simulink model "sampleModel7293_pp_1_1_mu"  (R2018a)
settings: Solver=VariableStepAuto  StartTime=0.0  StopTime=10.0  RelTol=1e-3
undefined symbols (not defined in the file): DiscIntNeverNeededParam
libraries: simulink x367
(part 1 of 13)
settings Model: Creator=cyfuzz  LastModifiedBy=shafiul
settings CodeAppCC: StateflowObjectComments=on

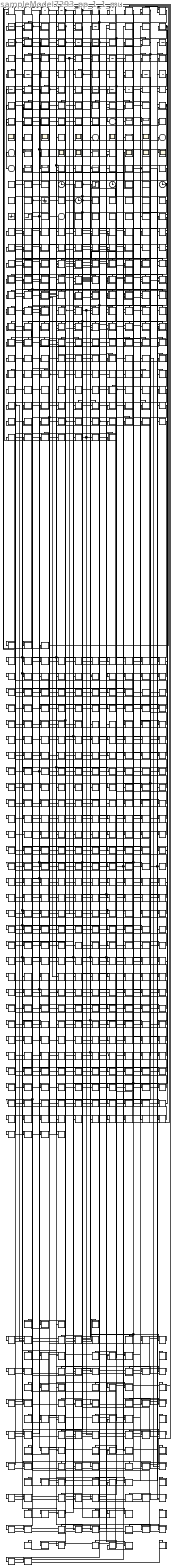
== system sampleModel7293_pp_1_1_mu ==
  cfblk134 : Inport
  cfblk{1,59..60,67} (4 alike) : simulink/Continuous/PID Controller (2DOF)  Controller=PID  TimeDomain=Discrete-time  SampleTime=1  IntegratorMethod=Forward Euler  FilterMethod=Forward Euler  Form=Parallel  UseFilter=on  ControllerParametersSource=internal  P=1  I=1  D=0  N=100  b=1  c=1  InitialConditionSource=internal  InitialConditionForIntegrator=0  InitialConditionForFilter=0  ExternalReset=none  LimitOutput=off  UpperSaturationLimit=inf  LowerSaturationLimit=-inf  LinearizeAsGain=off  AntiWindupMode=none  Kb=1  TrackingMode=off  Kt=1  PParamMin=[]  PParamMax=[]  IParamMin=[]  IParamMax=[]  DParamMin=[]  DParamMax=[]  NParamMin=[]  NParamMax=[]  bParamMin=[]  bParamMax=[]  cParamMin=[]  cParamMax=[]  KbParamMin=[]  KbParamMax=[]  KtParamMin=[]  KtParamMax=[]  POutMin=[]  POutMax=[]  IOutMin=[]  IOutMax=[]  DOutMin=[]  DOutMax=[]  NOutMin=[]  NOutMax=[]  bOutMin=[]  bOutMax=[]  cOutMin=[]  cOutMax=[]  KbOutMin=[]  KbOutMax=[]  KtOutMin=[]  KtOutMax=[]  IntegratorOutMin=[]  IntegratorOutMax=[]  FilterOutMin=[]  FilterOutMax=[]  SumOutMin=[]  SumOutMax=[]  Sum1OutMin=[]  Sum1OutMax=[]  Sum2OutMin=[]  Sum2OutMax=[]  Sum3OutMin=[]  Sum3OutMax=[]  SumI1OutMin=[]  SumI1OutMax=[]  SumI2OutMin=[]  SumI2OutMax=[]  SumI3OutMin=[]  SumI3OutMax=[]  SumDOutMin=[]  SumDOutMax=[]  SaturationOutMin=[]  SaturationOutMax=[]  IntegratorContinuousStateAttributes=''  IntegratorStateMustResolveToSignalObject=off  IntegratorRTWStateStorageClass=Auto  FilterContinuousStateAttributes=''  FilterStateMustResolveToSignalObject=off  FilterRTWStateStorageClass=Auto  DifferentiatorICPrevScaledInput=0  DifferentiatorOutMin=[]  DifferentiatorOutMax=[]  FilterDiffOutCoefMin=[]  FilterDiffOutCoefMax=[]  SumDenOutMin=[]  SumDenOutMax=[]  SumNumOutMin=[]  SumNumOutMax=[]  ReciprocalOutMin=[]  ReciprocalOutMax=[]  DivideOutMin=[]  DivideOutMax=[]  TunerSelectOption=Transfer Function Based (PID Tuner App)
  cfblk{10,15,35,48,54,70,73} (7 alike) : Delay  ShowEnablePort=on  SampleTime=1
      settings: InputPortMap=u0,e6
  cfblk{81,83,85,87,89,94..95,98..100} (10 alike) : Scope
      cfblk81 settings: Floating=on
      cfblk83 settings: Floating=on
      cfblk85 settings: Floating=on
      cfblk87 settings: Floating=on
      cfblk89 settings: Floating=on
      cfblk94 settings: Floating=on
      cfblk95 settings: Floating=on
      cfblk99 settings: Floating=on
  cfblk{78..79,88,92,96,102..103,106} (8 alike) : Display
  cfblk104 : simulink/Sinks/XY Graph  xmin=-1  xmax=1  ymin=-1  ymax=1  st=-1
  cfblk105 : ToWorkspace  VariableName=oefgltt  SaveFormat=Timeseries  SampleTime=-1
  cfblk107 : ToWorkspace  VariableName=romnstx  SaveFormat=Timeseries  SampleTime=-1
  cfblk{108..109,129..130} (4 alike) : RandomNumber  SampleTime=0.1
  cfblk{11,21,26,56} (4 alike) : DiscreteFilter  SampleTime=1
  cfblk110 : simulink/Sources/Counter Limited  uplimit=7  tsamp=1
  cfblk111 : simulink/Sources/Counter Free-Running  NumBits=16  tsamp=1
  cfblk112 : simulink/Sources/Ramp  slope=1  start=0  InitialOutput=0
  cfblk113 : simulink/Sources/Repeating Sequence Interpolated  OutValues=[3 1 4 2 1].'  TimeValues=[0 0.1 0.5 0.6 1].'  LookUpMeth=Interpolation-Use End Values  tsamp=0.01  OutMin=[]  OutMax=[]  OutDataTypeStr=double  OutputDataTypeScalingMode=double  OutDataType=fixdt(0,8)  OutScaling=2^-10
  cfblk{114,117,120,125} (4 alike) : Clock
  cfblk115 : DigitalClock
  cfblk116 : Step  After=79  SampleTime=0
  cfblk118 : simulink/Sources/Counter Free-Running  NumBits=16  tsamp=1
  cfblk119 : simulink/Sources/Repeating Sequence  rep_seq_t=[0 2]  rep_seq_y=[0 2]
  cfblk12 : Subsystem  TreatAsAtomicUnit=on
  cfblk121 : simulink/Sources/Repeating Sequence Stair  OutValues=[3 1 4 2 1].'  tsamp=1  OutMin=[]  OutMax=[]  OutDataTypeStr=double  OutputDataTypeScalingMode=double  OutDataType=fixdt(0,8)  ConRadixGroup=Best Precision: Vector-wise  OutScaling=2^-12
  cfblk122 : Constant  Value=5474  OutDataTypeStr=double  SampleTime=1
  cfblk123 : Ground
  cfblk124 : simulink/Sources/Chirp Signal  f1=0.1  T=100  f2=1
  cfblk126 : Constant  Value=0696  OutDataTypeStr=double  SampleTime=1
  cfblk127 : simulink/Sources/Repeating Sequence Stair  OutValues=[3 1 4 2 1].'  tsamp=1  OutMin=[]  OutMax=[]  OutDataTypeStr=double  OutputDataTypeScalingMode=double  OutDataType=fixdt(0,8)  ConRadixGroup=Best Precision: Vector-wise  OutScaling=2^-12
  cfblk128 : SignalGenerator  Units=rad/sec
  cfblk{13,23,46,65,216..217,221..226,228..229,232,234..238,241..246,248..254,257..258,260..267,269..272} (47 alike) : Delay  SampleTime=1
  cfblk131 : Ground
  cfblk132 : Step  After=47  SampleTime=0
  cfblk133 : simulink/Sources/Counter Limited  uplimit=7  tsamp=1
  cfblk135 : simulink/Sources/Repeating Sequence Stair  OutValues=[3 1 4 2 1].'  tsamp=1  OutMin=[]  OutMax=[]  OutDataTypeStr=double  OutputDataTypeScalingMode=double  OutDataType=fixdt(0,8)  ConRadixGroup=Best Precision: Vector-wise  OutScaling=2^-12
  cfblk136 : simulink/Sources/Repeating Sequence Interpolated  OutValues=[3 1 4 2 1].'  TimeValues=[0 0.1 0.5 0.6 1].'  LookUpMeth=Interpolation-Use End Values  tsamp=0.01  OutMin=[]  OutMax=[]  OutDataTypeStr=double  OutputDataTypeScalingMode=double  OutDataType=fixdt(0,8)  OutScaling=2^-10
  cfblk137 : DigitalClock
  cfblk138 : simulink/Sources/Repeating Sequence Interpolated  OutValues=[3 1 4 2 1].'  TimeValues=[0 0.1 0.5 0.6 1].'  LookUpMeth=Interpolation-Use End Values  tsamp=0.01  OutMin=[]  OutMax=[]  OutDataTypeStr=double  OutputDataTypeScalingMode=double  OutDataType=fixdt(0,8)  OutScaling=2^-10
  cfblk{139..163} (25 alike) : If  SampleTime=1
  cfblk14 : DiscreteStateSpace
  cfblk{4,16,25,37,51} (5 alike) : DiscreteIntegrator  OutDataTypeStr=double  ICPrevOutput=DiscIntNeverNeededParam  ICPrevScaledInput=DiscIntNeverNeededParam
  cfblk164 : Subsystem  TreatAsAtomicUnit=on
  cfblk165 : Subsystem  TreatAsAtomicUnit=on
  cfblk166 : Subsystem  TreatAsAtomicUnit=on
  cfblk167 : Subsystem  TreatAsAtomicUnit=on
  cfblk168 : Subsystem  TreatAsAtomicUnit=on
  cfblk169 : Subsystem  TreatAsAtomicUnit=on
  cfblk{17,24,36,43..44,71} (6 alike) : Delay  DelayLengthSource=Input port  SampleTime=1
      settings: InputPortMap=u0,p1
  cfblk170 : Subsystem  TreatAsAtomicUnit=on
  cfblk171 : Subsystem  TreatAsAtomicUnit=on
  cfblk172 : Subsystem  TreatAsAtomicUnit=on
  cfblk173 : Subsystem  TreatAsAtomicUnit=on
  cfblk174 : Subsystem  TreatAsAtomicUnit=on
  cfblk175 : Subsystem  TreatAsAtomicUnit=on
  cfblk176 : Subsystem  TreatAsAtomicUnit=on
  cfblk177 : Subsystem  TreatAsAtomicUnit=on
  cfblk178 : Subsystem  TreatAsAtomicUnit=on
  cfblk179 : Subsystem  TreatAsAtomicUnit=on
  cfblk{18,34,47,69} (4 alike) : simulink/Continuous/PID Controller  Controller=PID  TimeDomain=Discrete-time  SampleTime=1  IntegratorMethod=Forward Euler  FilterMethod=Forward Euler  Form=Parallel  UseFilter=on  ControllerParametersSource=internal  P=1  I=1  D=0  N=100  InitialConditionSource=internal  InitialConditionForIntegrator=0  InitialConditionForFilter=0  ExternalReset=none  LimitOutput=off  UpperSaturationLimit=inf  LowerSaturationLimit=-inf  LinearizeAsGain=off  AntiWindupMode=none  Kb=1  TrackingMode=off  Kt=1  PParamMin=[]  PParamMax=[]  IParamMin=[]  IParamMax=[]  DParamMin=[]  DParamMax=[]  NParamMin=[]  NParamMax=[]  KbParamMin=[]  KbParamMax=[]  KtParamMin=[]  KtParamMax=[]  POutMin=[]  POutMax=[]  IOutMin=[]  IOutMax=[]  DOutMin=[]  DOutMax=[]  NOutMin=[]  NOutMax=[]  KbOutMin=[]  KbOutMax=[]  KtOutMin=[]  KtOutMax=[]  IntegratorOutMin=[]  IntegratorOutMax=[]  FilterOutMin=[]  FilterOutMax=[]  SumOutMin=[]  SumOutMax=[]  SumI1OutMin=[]  SumI1OutMax=[]  SumI2OutMin=[]  SumI2OutMax=[]  SumI3OutMin=[]  SumI3OutMax=[]  SumDOutMin=[]  SumDOutMax=[]  SaturationOutMin=[]  SaturationOutMax=[]  IntegratorContinuousStateAttributes=''  IntegratorStateMustResolveToSignalObject=off  IntegratorRTWStateStorageClass=Auto  FilterContinuousStateAttributes=''  FilterStateMustResolveToSignalObject=off  FilterRTWStateStorageClass=Auto  DifferentiatorICPrevScaledInput=0  DifferentiatorOutMin=[]  DifferentiatorOutMax=[]  FilterDiffOutCoefMin=[]  FilterDiffOutCoefMax=[]  SumDenOutMin=[]  SumDenOutMax=[]  SumNumOutMin=[]  SumNumOutMax=[]  ReciprocalOutMin=[]  ReciprocalOutMax=[]  DivideOutMin=[]  DivideOutMax=[]  TunerSelectOption=Transfer Function Based (PID Tuner App)
  cfblk180 : Subsystem  TreatAsAtomicUnit=on
  cfblk181 : Subsystem  TreatAsAtomicUnit=on
  cfblk182 : Subsystem  TreatAsAtomicUnit=on
  cfblk183 : Subsystem  TreatAsAtomicUnit=on
  cfblk184 : Subsystem  TreatAsAtomicUnit=on
  cfblk185 : Subsystem  TreatAsAtomicUnit=on
  cfblk186 : Subsystem  TreatAsAtomicUnit=on
  cfblk187 : Subsystem  TreatAsAtomicUnit=on
  cfblk188 : Subsystem  TreatAsAtomicUnit=on
  cfblk189 : Subsystem  TreatAsAtomicUnit=on
  cfblk19 : simulink/Discrete/Transfer Fcn Real Zero  ZeroZ=0.75  ICPrevInput=0.0  DoSatur=off
      settings: SourceProductName=Simulink  SourceProductBaseCode=SL
  cfblk190 : Subsystem  TreatAsAtomicUnit=on
  cfblk191 : Subsystem  TreatAsAtomicUnit=on
  cfblk192 : Subsystem  TreatAsAtomicUnit=on
  cfblk193 : Subsystem  TreatAsAtomicUnit=on
  cfblk194 : Subsystem  TreatAsAtomicUnit=on
  cfblk195 : Subsystem  TreatAsAtomicUnit=on
  cfblk196 : Subsystem  TreatAsAtomicUnit=on
  cfblk197 : Subsystem  TreatAsAtomicUnit=on
  cfblk198 : Subsystem  TreatAsAtomicUnit=on
  cfblk199 : Subsystem  TreatAsAtomicUnit=on
  cfblk2 : Subsystem  TreatAsAtomicUnit=on
  cfblk20 : simulink/Discrete/Transfer Fcn First Order  PoleZ=0.95  ICPrevOutput=0.0  DoSatur=off
      settings: SourceProductName=Simulink
  cfblk200 : Subsystem  TreatAsAtomicUnit=on
  cfblk201 : Subsystem  TreatAsAtomicUnit=on
  cfblk202 : Subsystem  TreatAsAtomicUnit=on
  cfblk203 : Subsystem  TreatAsAtomicUnit=on
  cfblk204 : Subsystem  TreatAsAtomicUnit=on
  cfblk205 : Subsystem  TreatAsAtomicUnit=on
  cfblk206 : Subsystem  TreatAsAtomicUnit=on
  cfblk207 : Subsystem  TreatAsAtomicUnit=on
  cfblk208 : Subsystem  TreatAsAtomicUnit=on
  cfblk209 : Subsystem  TreatAsAtomicUnit=on
  cfblk210 : Subsystem  TreatAsAtomicUnit=on
  cfblk211 : Subsystem  TreatAsAtomicUnit=on
  cfblk212 : Subsystem  TreatAsAtomicUnit=on
  cfblk213 : Subsystem  TreatAsAtomicUnit=on
  cfblk214 : Subsystem  TreatAsAtomicUnit=on
  cfblk215 : Subsystem  TreatAsAtomicUnit=on
  cfblk218 : Subsystem  TreatAsAtomicUnit=on
  cfblk219 : Subsystem  TreatAsAtomicUnit=on
  cfblk22 : Subsystem  TreatAsAtomicUnit=on
  cfblk220 : Subsystem  TreatAsAtomicUnit=on
  cfblk227 : Subsystem  TreatAsAtomicUnit=on
  cfblk230 : Subsystem  TreatAsAtomicUnit=on
  cfblk231 : Subsystem  TreatAsAtomicUnit=on
  cfblk233 : Subsystem  TreatAsAtomicUnit=on
  cfblk239 : Subsystem  TreatAsAtomicUnit=on
  cfblk240 : Subsystem  TreatAsAtomicUnit=on
  cfblk247 : Subsystem  TreatAsAtomicUnit=on
  cfblk255 : Subsystem  TreatAsAtomicUnit=on
  cfblk256 : Subsystem  TreatAsAtomicUnit=on
  cfblk259 : Subsystem  TreatAsAtomicUnit=on
  cfblk268 : Subsystem  TreatAsAtomicUnit=on
  cfblk27 : DiscreteZeroPole  Poles=[0 0.5]  Gain=1
  cfblk273 : Subsystem  TreatAsAtomicUnit=on
  cfblk274 : DataTypeConversion  OutDataTypeStr=double
  cfblk275 : DataTypeConversion  OutDataTypeStr=double
  cfblk276 : DataTypeConversion  OutDataTypeStr=double
  cfblk277 : Subsystem  TreatAsAtomicUnit=on
  cfblk28 : simulink/Discrete/Transfer Fcn Lead or Lag  PoleZ=0.95  ZeroZ=0.75  ICPrevOutput=0.0  ICPrevInput=0.0  DoSatur=off
      settings: SourceProductName=Simulink  SourceProductBaseCode=SL
  cfblk29 : Subsystem  TreatAsAtomicUnit=on
  cfblk{3,7,50,58} (4 alike) : UnitDelay
  cfblk{30,42,49,57} (4 alike) : DiscreteTransferFcn  SampleTime=1
  cfblk31 : simulink/Discrete/Transfer Fcn Lead or Lag  PoleZ=0.95  ZeroZ=0.75  ICPrevOutput=0.0  ICPrevInput=0.0  DoSatur=off
      settings: SourceProductName=Simulink  SourceProductBaseCode=SL
  cfblk32 : Subsystem  TreatAsAtomicUnit=on
  cfblk33 : Subsystem  TreatAsAtomicUnit=on
  cfblk38 : DiscreteStateSpace
  cfblk39 : Subsystem  TreatAsAtomicUnit=on
  cfblk40 : Subsystem  TreatAsAtomicUnit=on
  cfblk41 : Subsystem  TreatAsAtomicUnit=on
  cfblk45 : Subsystem  TreatAsAtomicUnit=on
  cfblk5 : DiscreteStateSpace
  cfblk52 : Subsystem  TreatAsAtomicUnit=on
  cfblk53 : Subsystem  TreatAsAtomicUnit=on
  cfblk55 : simulink/Discrete/Difference  ICPrevInput=0.0  OutMin=[]  OutMax=[]  OutDataTypeStr=uint16  OutputDataTypeScalingMode=uint16  OutDataType=fixdt(1, 16)  OutScaling=2^-10  DoSatur=off
  cfblk6 : Subsystem  TreatAsAtomicUnit=on
  cfblk61 : simulink/Discrete/Transfer Fcn First Order  PoleZ=0.95  ICPrevOutput=0.0  DoSatur=off
      settings: SourceProductName=Simulink
  cfblk62 : Subsystem  TreatAsAtomicUnit=on
  cfblk63 : DiscreteZeroPole  Poles=[0 0.5]  Gain=1
  cfblk64 : Subsystem  TreatAsAtomicUnit=on
  cfblk66 : Subsystem  TreatAsAtomicUnit=on
  cfblk68 : Subsystem  TreatAsAtomicUnit=on
  cfblk72 : DiscreteFir  SampleTime=1
  cfblk74 : simulink/Discrete/Transfer Fcn Lead or Lag  PoleZ=0.95  ZeroZ=0.75  ICPrevOutput=0.0  ICPrevInput=0.0  DoSatur=off
      settings: SourceProductName=Simulink  SourceProductBaseCode=SL
  cfblk75 : ToWorkspace  VariableName=ullrodg  SaveFormat=Timeseries  SampleTime=-1
  cfblk76 : ToWorkspace  VariableName=mkrtbsh  SaveFormat=Timeseries  SampleTime=-1
  cfblk8 : Subsystem  TreatAsAtomicUnit=on
  cfblk80 : simulink/Sinks/XY Graph  xmin=-1  xmax=1  ymin=-1  ymax=1  st=-1
  cfblk82 : ToWorkspace  VariableName=zkrfoih  SaveFormat=Timeseries  SampleTime=-1
  cfblk84 : ToWorkspace  VariableName=gyvlriy  SaveFormat=Timeseries  SampleTime=-1
  cfblk9 : Subsystem  TreatAsAtomicUnit=on
  cfblk93 : ToWorkspace  VariableName=prwgbar  SaveFormat=Timeseries  SampleTime=-1
  cfblk97 : simulink/Sinks/XY Graph  xmin=-1  xmax=1  ymin=-1  ymax=1  st=-1
  cyemi_{0..37,39,41..42,51..55,95,104,160,168..169,181..184,242,278,288,321,329..330,369..373,381..384,393..394,404..406,419..423,463,474..475,515..517,527,585..590,626..629,633..635,670..673,680..682,727..728,770,781..783,791..792,794,870,878..879,916..918,949..950,1001..1002,1090,1142..1144,1180,1195,1210,1251..1252,1261..1263,1272..1274,1305..1306,1311..1312,1327,1367..1370,1406,1411..1413,1422..1423,1468..1511,1513..1534,1536,1538,1540..1548,1550..1577,1579..1598,1600..1605,1607..1614} (295 alike) : DataTypeConversion  OutDataTypeStr=double
  cyemi_{38,40,771,1512,1537,1549,1578,1599,1606} (9 alike) : DataTypeConversion  OutDataTypeStr=uint16
  cyemi_1535 : DataTypeConversion  OutDataTypeStr=uint8
  cyemi_1539 : DataTypeConversion  OutDataTypeStr=fixdt('ufix16_E3')
  cyemi_793 : DataTypeConversion  OutDataTypeStr=uint8
  emi_1010 : Subsystem  TreatAsAtomicUnit=on
  emi_{47,269,333,377,440,462,469,664,707,715,743,757,807,872,886,935,949,1012,1040,1111,1249,1298,1341,1397,1447,1519,1746,1790,1818,1882,1917,2016} (32 alike) : If  IfExpression=0 <= u1
  emi_{48,148,270,334,378,406,441,463,470,485,665,708,744,758,808,873,887,936,950,1013,1041,1112,1250,1299,1342,1398,1448,1484,1520,1548,1747,1791,1819,1883,1918,2017} (36 alike) : DataTypeConversion  OutDataTypeStr=double
  emi_1038 : Subsystem  TreatAsAtomicUnit=on
  emi_1109 : Subsystem  TreatAsAtomicUnit=on
  emi_1247 : Subsystem  TreatAsAtomicUnit=on
  emi_1296 : Subsystem  TreatAsAtomicUnit=on
  emi_1339 : Subsystem  TreatAsAtomicUnit=on
  emi_1395 : Subsystem  TreatAsAtomicUnit=on
  emi_1445 : Subsystem  TreatAsAtomicUnit=on
  emi_145 : Subsystem  TreatAsAtomicUnit=on
  emi_147 : If  IfExpression=-8.861719e+01 <= u1
  emi_1481 : Subsystem  TreatAsAtomicUnit=on
  emi_1483 : If  IfExpression=-2.482843e+00 <= u1  SampleTime=1
  emi_1517 : Subsystem  TreatAsAtomicUnit=on
  emi_1545 : Subsystem  TreatAsAtomicUnit=on
  emi_1547 : If  IfExpression=-7.093048e-01 <= u1
  emi_1744 : Subsystem  TreatAsAtomicUnit=on
  emi_1788 : Subsystem  TreatAsAtomicUnit=on
  emi_1816 : Subsystem  TreatAsAtomicUnit=on
  emi_1880 : Subsystem  TreatAsAtomicUnit=on
  emi_1915 : Subsystem  TreatAsAtomicUnit=on
  emi_2014 : Subsystem  TreatAsAtomicUnit=on
  emi_267 : Subsystem  TreatAsAtomicUnit=on
  emi_331 : Subsystem  TreatAsAtomicUnit=on
  emi_375 : Subsystem  TreatAsAtomicUnit=on
  emi_403 : Subsystem  TreatAsAtomicUnit=on
  emi_405 : If  IfExpression=-2.482843e+00 <= u1  SampleTime=1
  emi_438 : Subsystem  TreatAsAtomicUnit=on
  emi_45 : Subsystem  TreatAsAtomicUnit=on
  emi_460 : Subsystem  TreatAsAtomicUnit=on
  emi_467 : Subsystem  TreatAsAtomicUnit=on
  emi_482 : Subsystem  TreatAsAtomicUnit=on
  emi_484 : If  IfExpression=5474 <= u1
  emi_662 : Subsystem  TreatAsAtomicUnit=on
  emi_705 : Subsystem  TreatAsAtomicUnit=on
  emi_713 : Subsystem  TreatAsAtomicUnit=on
  emi_716 : DataTypeConversion  OutDataTypeStr=uint16
  emi_741 : Subsystem  TreatAsAtomicUnit=on
  emi_755 : Subsystem  TreatAsAtomicUnit=on
  emi_805 : Subsystem  TreatAsAtomicUnit=on
  emi_870 : Subsystem  TreatAsAtomicUnit=on
  emi_884 : Subsystem  TreatAsAtomicUnit=on
  emi_933 : Subsystem  TreatAsAtomicUnit=on
  emi_947 : Subsystem  TreatAsAtomicUnit=on
  cfblk77 : Outport
  cfblk86 : Outport  Port=2
  cfblk90 : Outport  Port=3
  cfblk91 : Outport  Port=4
  cfblk101 : Outport  Port=5
  wires:
  cfblk123/1 -> cfblk78/1, cyemi_1582/1
  cfblk119/1 -> cyemi_1545/1, cyemi_1583/1
  cfblk112/1 -> cfblk104/1
  cfblk13/1 -> cfblk103/1
  cfblk14/1 -> cyemi_24/1, cyemi_1614/1
  cfblk34/1 -> cyemi_393/1, cyemi_1475/1
  cfblk43/1 -> cfblk101/1
  cfblk5/1 -> cfblk77/1, cyemi_1274/1
  cfblk202/1(cfblk2) -> cyemi_1472/1, cyemi_1561/1
  cfblk20/1 -> cyemi_1485/1, cyemi_1487/1, cyemi_1550/1
  cfblk55/1 -> cyemi_1549/1, cyemi_1599/1
  cfblk108/1 -> cyemi_1272/1, emi_1484/1, cfblk80/2
  cfblk44/1 -> cfblk92/1
  cfblk31/1 -> cyemi_18/1, cyemi_1576/1
  cfblk24/1 -> cyemi_34/1, cyemi_1546/1
  cfblk194/1(cfblk2) -> cyemi_728/1, cyemi_1504/1
  cfblk196/1(cfblk2) -> cyemi_1195/1, cyemi_1604/1
  cfblk137/1 -> cyemi_1541/1, cyemi_1607/1
  cfblk164/2(cfblk13) -> cfblk90/1
  cfblk11/1 -> cyemi_1510/1, emi_1520/1, cyemi_1477/1, cyemi_1478/1
  cfblk26/1 -> cyemi_1470/1, cyemi_1530/1, cyemi_628/1
  cfblk128/1 -> cfblk98/1
  cfblk127/1 -> cfblk86/1
  cfblk61/1 -> cfblk79/1
  cfblk18/1 -> cyemi_682/1, cyemi_1367/1
  cfblk42/1 -> cyemi_1529/1, cyemi_1611/1
  cfblk49/1 -> cyemi_1497/1, cyemi_1612/1
  cfblk166/2(cfblk11) -> cfblk97/1
  cfblk165/1(cfblk2) -> cfblk88/1
  cfblk30/1 -> cyemi_55/1, cyemi_168/1
  cfblk176/1(cfblk2) -> cfblk102/1
  cfblk4/1 -> cyemi_278/1, emi_1548/1, cyemi_1581/1
  cfblk179/2(cfblk13) -> cfblk104/2
  cfblk174/2(cfblk9) -> cyemi_1370/1, cyemi_1522/1
  cfblk126/1 -> cyemi_372/1, cyemi_1251/1
  cfblk37/1 -> cyemi_1500/1, cyemi_1503/1
  cfblk58/1 -> cyemi_169/1, cyemi_1552/1
  cfblk28/1 -> cyemi_383/1, cyemi_1563/1
  cfblk212/1(cfblk2) -> cfblk96/1, cfblk91/1
  cfblk125/1 -> cyemi_242/1, cyemi_588/1, cyemi_627/1
  cfblk166/3(cfblk12) -> cyemi_53/1, cyemi_1210/1
  cfblk204/3(cfblk13) -> cyemi_1506/1, cyemi_1508/1, cyemi_1589/1
  cfblk195/1(cfblk2) -> cyemi_1369/1, cyemi_1476/1
  cfblk21/1 -> cyemi_10/1, emi_378/1, cyemi_589/1
  cfblk183/4(cfblk14) -> cyemi_1513/1, cyemi_1514/1
  cfblk181/2(cfblk9) -> cfblk80/1
  cfblk175/5(cfblk15) -> cfblk97/2
  cfblk23/1 -> cfblk106/1, emi_665/1
  cfblk197/2(cfblk15) -> cyemi_1532/1, cyemi_1605/1
  cfblk188/2(cfblk12) -> cyemi_629/1, cyemi_1483/1, cyemi_1480/1
  cfblk115/1 -> cyemi_516/1, cyemi_586/1
  cfblk120/1 -> cyemi_404/1, cyemi_463/1
  cfblk139/1 -> cfblk164/Action
  cfblk139/2 -> cfblk165/Action
  cfblk140/1 -> cfblk166/Action
  cfblk140/2 -> cfblk167/Action
  cfblk141/1 -> cfblk168/Action
  cfblk141/2 -> cfblk169/Action
  cfblk142/1 -> cfblk170/Action
  cfblk142/2 -> cfblk171/Action
  cfblk143/1 -> cfblk172/Action
  cfblk143/2 -> cfblk173/Action
  cfblk144/1 -> cfblk174/Action
  cfblk144/2 -> cfblk175/Action
  cfblk145/1 -> cfblk176/Action
  cfblk145/2 -> cfblk177/Action
  cfblk146/1 -> cfblk178/Action
  cfblk146/2 -> cfblk179/Action
  cfblk147/1 -> cfblk180/Action
  cfblk147/2 -> cfblk181/Action
  cfblk148/1 -> cfblk182/Action
  cfblk148/2 -> cfblk183/Action
  cfblk149/1 -> cfblk184/Action
  cfblk149/2 -> cfblk185/Action
  cfblk150/1 -> cfblk186/Action
  cfblk150/2 -> cfblk187/Action
  cfblk151/1 -> cfblk188/Action
  cfblk151/2 -> cfblk189/Action
  cfblk152/1 -> cfblk190/Action
  cfblk152/2 -> cfblk191/Action
  cfblk153/1 -> cfblk192/Action
  cfblk153/2 -> cfblk193/Action
  cfblk154/1 -> cfblk194/Action
  cfblk154/2 -> cfblk195/Action
  cfblk155/1 -> cfblk196/Action
  cfblk155/2 -> cfblk197/Action
  cfblk156/1 -> cfblk198/Action
  cfblk156/2 -> cfblk199/Action
  cfblk157/1 -> cfblk200/Action
  cfblk157/2 -> cfblk201/Action
  cfblk158/1 -> cfblk202/Action
  cfblk158/2 -> cfblk203/Action
  cfblk159/1 -> cfblk204/Action
  cfblk159/2 -> cfblk205/Action
  cfblk160/1 -> cfblk206/Action
  cfblk160/2 -> cfblk207/Action
  cfblk161/1 -> cfblk208/Action
  cfblk161/2 -> cfblk209/Action
  cfblk162/1 -> cfblk210/Action
  cfblk162/2 -> cfblk211/Action
  cfblk163/1 -> cfblk212/Action
  cfblk163/2 -> cfblk213/Action
  cyemi_0/1 -> cfblk1/1
  cfblk264/1 -> cyemi_0/1, emi_463/1
  cyemi_1/1 -> cfblk1/2
  cfblk117/1 -> cyemi_1/1
  cyemi_2/1 -> cfblk10/1
  cfblk3/1 -> cyemi_2/1, emi_470/1
  cyemi_3/1 -> cfblk10/2
  cfblk204/1(cfblk2) -> cyemi_3/1
  cyemi_4/1 -> cfblk105/1
  cyemi_5/1 -> cfblk107/1
  cfblk193/1(cfblk2) -> cyemi_5/1
  cyemi_6/1 -> cfblk11/1
  cfblk183/1(cfblk2) -> cyemi_6/1
  cfblk1/1 -> cyemi_8/1
  cyemi_9/1 -> cfblk13/1
  cfblk210/1(cfblk2) -> cyemi_9/1
  cyemi_10/1 -> cfblk139/1
  cyemi_11/1 -> cfblk14/1
  cyemi_12/1 -> cfblk140/1
  cfblk192/1(cfblk2) -> cyemi_12/1
  cyemi_13/1 -> cfblk141/1
  cfblk262/1 -> cyemi_13/1
  cyemi_14/1 -> cfblk142/1
  cfblk122/1 -> cyemi_14/1, emi_485/1
  cyemi_15/1 -> cfblk143/1
  cfblk132/1 -> cyemi_15/1, emi_48/1
  cyemi_16/1 -> cfblk144/1
  cfblk36/1 -> cyemi_16/1
  cyemi_17/1 -> cfblk145/1
  cfblk272/1 -> cyemi_17/1
  cyemi_18/1 -> cfblk146/1
  cyemi_19/1 -> cfblk147/1
  cfblk217/1 -> cyemi_19/1
  cyemi_20/1 -> cfblk148/1
  cfblk48/1 -> cyemi_20/1
  cyemi_21/1 -> cfblk149/1
  cfblk246/1 -> cyemi_21/1
  cyemi_22/1 -> cfblk15/1
  cfblk56/1 -> cyemi_22/1
  cyemi_23/1 -> cfblk15/2
  cyemi_24/1 -> cfblk150/1
  cyemi_25/1 -> cfblk151/1
  cfblk203/1(cfblk2) -> cyemi_25/1
  cyemi_26/1 -> cfblk152/1
  cfblk201/1(cfblk2) -> cyemi_26/1
  cyemi_27/1 -> cfblk153/1
  cyemi_28/1 -> cfblk154/1
  cfblk238/1 -> cyemi_28/1
  cyemi_29/1 -> cfblk155/1
  cfblk261/1 -> cyemi_29/1
  cyemi_30/1 -> cfblk156/1
  cfblk241/1 -> cyemi_30/1
  cyemi_31/1 -> cfblk157/1
  cfblk198/1(cfblk2) -> cyemi_31/1
  cyemi_32/1 -> cfblk158/1
  cfblk109/1 -> cyemi_32/1, emi_406/1
  cyemi_33/1 -> cfblk159/1
  cfblk251/1 -> cyemi_33/1, emi_148/1
  cyemi_34/1 -> cfblk16/1
  cyemi_35/1 -> cfblk160/1
  cfblk190/2(cfblk7) -> cyemi_35/1
  cyemi_36/1 -> cfblk161/1
  cyemi_37/1 -> cfblk162/1
  cfblk136/1 -> cyemi_37/1
  cyemi_38/1 -> cfblk163/1
  cfblk164/1(cfblk2) -> cyemi_38/1
  cyemi_39/1 -> cfblk164/1(cfblk1)
  cfblk223/1 -> cyemi_39/1, emi_1747/1
  cyemi_40/1 -> cfblk164/2(cfblk10)
  cfblk252/1 -> cyemi_40/1
  cyemi_41/1 -> cfblk164/3(cfblk11)
  cfblk180/1(cfblk2) -> cyemi_41/1
  cyemi_42/1 -> cfblk164/4(cfblk12)
  cyemi_51/1 -> cfblk165/1(cfblk1)
  cfblk226/1 -> cyemi_51/1
  cyemi_52/1 -> cfblk165/2(cfblk10)
  cfblk267/1 -> cyemi_52/1
  cyemi_53/1 -> cfblk165/3(cfblk11)
  cyemi_54/1 -> cfblk165/4(cfblk12)
  cfblk254/1 -> cyemi_54/1
  cyemi_55/1 -> cfblk165/5(cfblk13)
  cyemi_95/1 -> cfblk166/1(cfblk1)
  cyemi_104/1 -> cfblk167/1(cfblk1)
  cfblk216/1 -> cyemi_104/1
  cyemi_160/1 -> cfblk168/1(cfblk1)
  cfblk228/1 -> cyemi_160/1, emi_1883/1
  cyemi_168/1 -> cfblk169/1(cfblk1)
  cyemi_169/1 -> cfblk169/2(cfblk12)
  cyemi_181/1 -> cfblk17/1
  cfblk211/3(cfblk7) -> cyemi_181/1
  cyemi_182/1 -> cfblk17/2
  cfblk186/2(cfblk8) -> cyemi_182/1
  cyemi_183/1 -> cfblk170/1(cfblk1)
  cfblk171/2(cfblk9) -> cyemi_183/1
  cyemi_184/1 -> cfblk170/2(cfblk11)
  cfblk189/2(cfblk14) -> cyemi_184/1
  cyemi_242/1 -> cfblk171/1(cfblk1)
  cyemi_278/1 -> cfblk172/1(cfblk1)
  cyemi_288/1 -> cfblk173/1(cfblk1)
  cfblk73/1 -> cyemi_288/1
  cyemi_321/1 -> cfblk174/1(cfblk1)
  cfblk182/1(cfblk2) -> cyemi_321/1
  cyemi_329/1 -> cfblk175/1(cfblk1)
  cyemi_330/1 -> cfblk175/2(cfblk11)
  cfblk235/1 -> cyemi_330/1
  cyemi_369/1 -> cfblk176/1(cfblk1)
  cyemi_370/1 -> cfblk176/2(cfblk8)
  cfblk248/1 -> cyemi_370/1
  cyemi_371/1 -> cfblk176/3(cfblk9)
  cfblk270/1 -> cyemi_371/1
  cyemi_372/1 -> cfblk176/4(cfblk10)
  cyemi_373/1 -> cfblk176/5(cfblk11)
  cfblk263/1 -> cyemi_373/1
  cyemi_381/1 -> cfblk177/1(cfblk1)
  cfblk237/1 -> cyemi_381/1
  cyemi_382/1 -> cfblk177/2(cfblk9)
  cyemi_383/1 -> cfblk177/3(cfblk10)
  cyemi_384/1 -> cfblk177/4(cfblk11)
  cfblk269/1 -> cyemi_384/1
  cyemi_393/1 -> cfblk178/1(cfblk1)
  cyemi_394/1 -> cfblk178/2(cfblk11)
  cfblk57/1 -> cyemi_394/1
  cyemi_404/1 -> cfblk179/1(cfblk1)
  cyemi_405/1 -> cfblk179/2(cfblk11)
  cfblk232/1 -> cyemi_405/1, emi_950/1
  cyemi_406/1 -> cfblk179/3(cfblk12)
  cyemi_419/1 -> cfblk18/1
  cfblk51/1 -> cyemi_419/1
  cyemi_420/1 -> cfblk180/1(cfblk1)
  cfblk189/1(cfblk2) -> cyemi_420/1
  cyemi_421/1 -> cfblk180/2(cfblk14)
  cfblk253/1 -> cyemi_421/1, emi_1342/1
  cyemi_422/1 -> cfblk180/3(cfblk15)
  cfblk208/2(cfblk13) -> cyemi_422/1
  cyemi_423/1 -> cfblk180/4(cfblk16)
  cfblk167/3(cfblk16) -> cyemi_423/1
  cyemi_463/1 -> cfblk181/1(cfblk1)
  cyemi_474/1 -> cfblk182/1(cfblk1)
  cfblk172/1(cfblk2) -> cyemi_474/1
  cyemi_475/1 -> cfblk182/2(cfblk11)
  cfblk205/3(cfblk12) -> cyemi_475/1
  cyemi_515/1 -> cfblk183/1(cfblk1)
  cyemi_516/1 -> cfblk183/2(cfblk10)
  cyemi_517/1 -> cfblk183/3(cfblk11)
  cyemi_527/1 -> cfblk184/1(cfblk1)
  cfblk175/1(cfblk2) -> cyemi_527/1
  cyemi_585/1 -> cfblk185/1(cfblk1)
  cyemi_586/1 -> cfblk185/2(cfblk12)
  cyemi_587/1 -> cfblk185/3(cfblk13)
  cyemi_588/1 -> cfblk185/4(cfblk14)
  cyemi_589/1 -> cfblk185/5(cfblk15)
  cyemi_590/1 -> cfblk185/6(cfblk16)
  cfblk250/1 -> cyemi_590/1
  cyemi_626/1 -> cfblk186/1(cfblk1)
  cfblk206/3(cfblk14) -> cyemi_626/1
  cyemi_627/1 -> cfblk186/2(cfblk5)
  cyemi_628/1 -> cfblk186/3(cfblk6)
  cyemi_629/1 -> cfblk186/4(cfblk7)
  cyemi_633/1 -> cfblk187/1(cfblk1)
  cfblk124/1 -> cyemi_633/1
  cyemi_634/1 -> cfblk187/2(cfblk8)
  cfblk175/2(cfblk12) -> cyemi_634/1
  cyemi_635/1 -> cfblk187/3(cfblk9)
  cfblk169/3(cfblk14) -> cyemi_635/1
  cyemi_670/1 -> cfblk188/1(cfblk1)
  cfblk266/1 -> cyemi_670/1, emi_1299/1
  cyemi_671/1 -> cfblk188/2(cfblk9)
  cyemi_672/1 -> cfblk188/3(cfblk10)
  cyemi_673/1 -> cfblk188/4(cfblk11)
  cfblk222/1 -> cyemi_673/1
  cyemi_680/1 -> cfblk189/1(cfblk1)
  cfblk229/1 -> cyemi_680/1, emi_1250/1
  cyemi_681/1 -> cfblk189/2(cfblk12)
  cfblk167/2(cfblk15) -> cyemi_681/1
  cyemi_682/1 -> cfblk189/3(cfblk13)
  cyemi_727/1 -> cfblk19/1
  cfblk169/1(cfblk2) -> cyemi_727/1
  cyemi_728/1 -> cfblk190/1(cfblk1)
  cyemi_770/1 -> cfblk191/1(cfblk1)
  cyemi_771/1 -> cfblk191/2(cfblk8)
  cfblk70/1 -> cyemi_771/1, emi_716/1
  cyemi_781/1 -> cfblk192/1(cfblk1)
  cfblk243/1 -> cyemi_781/1
  cyemi_782/1 -> cfblk192/2(cfblk9)
  cfblk221/1 -> cyemi_782/1
  cyemi_783/1 -> cfblk192/3(cfblk10)
  cfblk258/1 -> cyemi_783/1
  cyemi_791/1 -> cfblk193/1(cfblk1)
  cfblk129/1 -> cyemi_791/1
  cyemi_792/1 -> cfblk193/2(cfblk13)
  cfblk271/1 -> cyemi_792/1
  cyemi_793/1 -> cfblk193/3(cfblk14)
  cfblk133/1 -> cyemi_793/1
  cyemi_794/1 -> cfblk193/4(cfblk15)
  cfblk50/1 -> cyemi_794/1, emi_1791/1
  cyemi_870/1 -> cfblk194/1(cfblk1)
  cfblk236/1 -> cyemi_870/1
  cyemi_878/1 -> cfblk195/1(cfblk1)
  cyemi_879/1 -> cfblk195/2(cfblk7)
  cfblk244/1 -> cyemi_879/1
  cyemi_916/1 -> cfblk196/1(cfblk1)
  cfblk131/1 -> cyemi_916/1
  cyemi_917/1 -> cfblk196/2(cfblk9)
  cyemi_918/1 -> cfblk196/3(cfblk10)
  cfblk260/1 -> cyemi_918/1, emi_441/1
  cyemi_949/1 -> cfblk197/1(cfblk1)
  cfblk192/2(cfblk11) -> cyemi_949/1
  cyemi_950/1 -> cfblk197/2(cfblk14)
  cfblk200/1(cfblk2) -> cyemi_950/1
  cyemi_1001/1 -> cfblk198/1(cfblk1)
  cfblk178/2(cfblk12) -> cyemi_1001/1
  cyemi_1002/1 -> cfblk198/2(cfblk13)
  cfblk242/1 -> cyemi_1002/1
  cyemi_1090/1 -> cfblk199/1(cfblk1)
  cfblk171/1(cfblk2) -> cyemi_1090/1
  cfblk177/2(cfblk12) -> cyemi_1142/1
  cyemi_1143/1 -> cfblk20/1
  cfblk60/1 -> cyemi_1143/1
  cyemi_1144/1 -> cfblk200/1(cfblk1)
  cyemi_1180/1 -> cfblk201/1(cfblk1)
  cfblk265/1 -> cyemi_1180/1
  cyemi_1195/1 -> cfblk202/1(cfblk1)
  cyemi_1210/1 -> cfblk203/1(cfblk1)
  cyemi_1251/1 -> cfblk204/1(cfblk1)
  cyemi_1252/1 -> cfblk204/2(cfblk11)
  cfblk245/1 -> cyemi_1252/1
  cyemi_1261/1 -> cfblk205/1(cfblk1)
  cyemi_1262/1 -> cfblk205/2(cfblk9)
  cfblk114/1 -> cyemi_1262/1, emi_1013/1
  cyemi_1263/1 -> cfblk205/3(cfblk10)
  cyemi_1272/1 -> cfblk206/1(cfblk1)
  cyemi_1273/1 -> cfblk206/2(cfblk11)
  cfblk210/2(cfblk16) -> cyemi_1273/1
  cyemi_1274/1 -> cfblk206/3(cfblk12)
  cyemi_1305/1 -> cfblk207/1(cfblk1)
  cfblk134/1 -> cyemi_1305/1
  cyemi_1306/1 -> cfblk207/2(cfblk7)
  cfblk211/2(cfblk6) -> cyemi_1306/1
  cyemi_1311/1 -> cfblk208/1(cfblk1)
  cyemi_1312/1 -> cfblk208/2(cfblk12)
  cfblk234/1 -> cyemi_1312/1
  cyemi_1327/1 -> cfblk209/1(cfblk1)
  cfblk249/1 -> cyemi_1327/1
  cyemi_1367/1 -> cfblk21/1
  cyemi_1368/1 -> cfblk210/1(cfblk1)
  cyemi_1369/1 -> cfblk210/2(cfblk14)
  cyemi_1370/1 -> cfblk210/3(cfblk15)
  cyemi_1406/1 -> cfblk211/1(cfblk1)
  cfblk190/1(cfblk2) -> cyemi_1406/1
  cyemi_1411/1 -> cfblk212/1(cfblk1)
  cfblk193/2(cfblk16) -> cyemi_1411/1
  cyemi_1412/1 -> cfblk212/2(cfblk8)
  cfblk177/3(cfblk13) -> cyemi_1412/1
  cyemi_1413/1 -> cfblk212/3(cfblk9)
  cfblk167/1(cfblk2) -> cyemi_1413/1
  cyemi_1422/1 -> cfblk213/1(cfblk1)
  cfblk25/1 -> cyemi_1422/1
  cyemi_1423/1 -> cfblk213/2(cfblk12)
  cfblk224/1 -> cyemi_1423/1
  cfblk19/1 -> cyemi_1468/1
  cfblk178/1(cfblk2) -> cyemi_1469/1
  cyemi_1470/1 -> cfblk216/1
  cyemi_1471/1 -> cfblk217/1
  cfblk15/1 -> cyemi_1471/1
  cfblk184/1(cfblk2) -> cyemi_1473/1
  cyemi_1477/1 -> cfblk221/1
  cyemi_1478/1 -> cfblk222/1
  cyemi_1479/1 -> cfblk223/1
  cyemi_1480/1 -> cfblk224/1
  cyemi_1481/1 -> cfblk225/1
  cfblk186/1(cfblk2) -> cyemi_1481/1
  cyemi_1482/1 -> cfblk226/1
  cfblk17/1 -> cyemi_1482/1
  cyemi_1484/1 -> cfblk228/1
  cfblk185/1(cfblk2) -> cyemi_1484/1
  cyemi_1485/1 -> cfblk229/1
  cyemi_1486/1 -> cfblk23/1
  cfblk205/2(cfblk11) -> cyemi_1486/1
  cfblk10/1 -> cyemi_1488/1
  cyemi_1489/1 -> cfblk232/1
  cfblk179/3(cfblk14) -> cyemi_1490/1
  cyemi_1491/1 -> cfblk234/1
  cfblk176/2(cfblk12) -> cyemi_1491/1
  cyemi_1492/1 -> cfblk235/1
  cfblk179/4(cfblk15) -> cyemi_1492/1
  cyemi_1493/1 -> cfblk236/1
  cfblk274/1 -> cyemi_1493/1
  cyemi_1494/1 -> cfblk237/1
  cfblk211/1(cfblk2) -> cyemi_1494/1
  cyemi_1495/1 -> cfblk238/1
  cfblk63/1 -> cyemi_1495/1
  cfblk206/2(cfblk13) -> cyemi_1496/1
  cyemi_1497/1 -> cfblk24/1
  cyemi_1498/1 -> cfblk24/2
  cfblk257/1 -> cyemi_1498/1
  cfblk206/4(cfblk15) -> cyemi_1499/1
  cyemi_1500/1 -> cfblk241/1
  cyemi_1501/1 -> cfblk242/1
  cfblk199/1(cfblk2) -> cyemi_1501/1
  cyemi_1502/1 -> cfblk243/1
  cfblk7/1 -> cyemi_1502/1
  cyemi_1503/1 -> cfblk244/1
  cyemi_1504/1 -> cfblk245/1
  cyemi_1505/1 -> cfblk246/1
  cfblk72/1 -> cyemi_1505/1
  cyemi_1507/1 -> cfblk248/1
  cyemi_1508/1 -> cfblk249/1
  cyemi_1509/1 -> cfblk25/1
  cfblk276/1 -> cyemi_1509/1, emi_1918/1
  cyemi_1510/1 -> cfblk250/1
  cyemi_1511/1 -> cfblk251/1
  cfblk67/1 -> cyemi_1511/1
  cyemi_1512/1 -> cfblk252/1
  cfblk191/1(cfblk2) -> cyemi_1512/1
  cyemi_1513/1 -> cfblk253/1
  cyemi_1514/1 -> cfblk254/1
  cfblk187/1(cfblk2) -> cyemi_1515/1
  cfblk187/2(cfblk10) -> cyemi_1516/1
  cyemi_1517/1 -> cfblk257/1
  cfblk175/3(cfblk13) -> cyemi_1517/1
  cyemi_1518/1 -> cfblk258/1
  cfblk175/4(cfblk14) -> cyemi_1518/1
  cfblk173/1(cfblk2) -> cyemi_1519/1
  cyemi_1520/1 -> cfblk26/1
  cfblk208/1(cfblk2) -> cyemi_1520/1
  cyemi_1521/1 -> cfblk260/1
  cfblk173/2(cfblk12) -> cyemi_1521/1
  cyemi_1522/1 -> cfblk261/1
  cyemi_1523/1 -> cfblk262/1
  cyemi_1524/1 -> cfblk263/1
  cyemi_1525/1 -> cfblk264/1
  cfblk16/1 -> cyemi_1525/1
  cyemi_1526/1 -> cfblk265/1
  cyemi_1527/1 -> cfblk266/1
  cfblk213/2(cfblk13) -> cyemi_1527/1
  cyemi_1528/1 -> cfblk267/1
  cfblk71/1 -> cyemi_1528/1
  cyemi_1530/1 -> cfblk269/1
  cyemi_1531/1 -> cfblk27/1
  cfblk121/1 -> cyemi_1531/1
  cyemi_1532/1 -> cfblk270/1
  cyemi_1533/1 -> cfblk271/1
  cfblk178/3(cfblk13) -> cyemi_1533/1
  cyemi_1534/1 -> cfblk272/1
  cfblk177/4(cfblk14) -> cyemi_1534/1
  cfblk110/1 -> cyemi_1535/1
  cyemi_1536/1 -> cfblk274/1
  cfblk47/1 -> cyemi_1536/1
  cyemi_1537/1 -> cfblk275/1
  cfblk35/1 -> cyemi_1537/1
  cyemi_1538/1 -> cfblk276/1
  cfblk69/1 -> cyemi_1538/1
  cfblk74/1 -> cyemi_1539/1
  cyemi_1540/1 -> cfblk28/1
  cfblk166/1(cfblk2) -> cyemi_1540/1
  cfblk59/1 -> cyemi_1542/1
  cyemi_1543/1 -> cfblk3/1
  cyemi_1544/1 -> cfblk30/1
  cfblk205/1(cfblk2) -> cyemi_1544/1
  cyemi_1545/1 -> cfblk31/1
  cfblk197/1(cfblk2) -> cyemi_1547/1
  cyemi_1548/1 -> cfblk34/1
  cfblk138/1 -> cyemi_1548/1
  cyemi_1549/1 -> cfblk35/1
  cyemi_1550/1 -> cfblk35/2
  cyemi_1551/1 -> cfblk36/1
  cyemi_1552/1 -> cfblk36/2
  cyemi_1553/1 -> cfblk37/1
  cfblk190/3(cfblk8) -> cyemi_1553/1
  cyemi_1554/1 -> cfblk38/1
  cfblk168/2(cfblk8) -> cyemi_1554/1
  cfblk188/1(cfblk2) -> cyemi_1555/1
  cyemi_1556/1 -> cfblk4/1
  cfblk130/1 -> cyemi_1556/1
  cfblk189/3(cfblk15) -> cyemi_1557/1
  cfblk179/1(cfblk2) -> cyemi_1558/1
  cyemi_1559/1 -> cfblk42/1
  cyemi_1560/1 -> cfblk43/1
  cfblk165/2(cfblk14) -> cyemi_1560/1
  cyemi_1561/1 -> cfblk43/2
  cyemi_1562/1 -> cfblk44/1
  cfblk181/1(cfblk2) -> cyemi_1562/1
  cyemi_1563/1 -> cfblk44/2
  cfblk183/3(cfblk13) -> cyemi_1564/1
  cyemi_1565/1 -> cfblk46/1
  cfblk135/1 -> cyemi_1565/1
  cyemi_1566/1 -> cfblk47/1
  cfblk275/1 -> cyemi_1566/1, emi_887/1
  cyemi_1567/1 -> cfblk48/1
  cfblk225/1 -> cyemi_1567/1, emi_334/1
  cyemi_1568/1 -> cfblk48/2
  cfblk168/1(cfblk2) -> cyemi_1568/1
  cyemi_1569/1 -> cfblk49/1
  cfblk213/1(cfblk2) -> cyemi_1569/1
  cyemi_1570/1 -> cfblk5/1
  cfblk172/2(cfblk10) -> cyemi_1570/1
  cyemi_1571/1 -> cfblk50/1
  cfblk116/1 -> cyemi_1571/1
  cyemi_1572/1 -> cfblk51/1
  cfblk65/1 -> cyemi_1572/1
  cfblk209/1(cfblk2) -> cyemi_1573/1
  cfblk170/3(cfblk13) -> cyemi_1574/1
  cfblk169/2(cfblk13) -> cyemi_1575/1
  cyemi_1576/1 -> cfblk54/1
  cyemi_1577/1 -> cfblk54/2
  cfblk170/1(cfblk2) -> cyemi_1577/1
  cyemi_1578/1 -> cfblk55/1
  cfblk118/1 -> cyemi_1578/1
  cyemi_1579/1 -> cfblk56/1
  cfblk174/1(cfblk2) -> cyemi_1579/1
  cyemi_1580/1 -> cfblk57/1
  cfblk177/1(cfblk2) -> cyemi_1580/1
  cyemi_1581/1 -> cfblk58/1
  cyemi_1582/1 -> cfblk59/1
  cyemi_1583/1 -> cfblk59/2
  cfblk170/2(cfblk12) -> cyemi_1584/1
  cyemi_1585/1 -> cfblk60/1
  cfblk46/1 -> cyemi_1585/1
  cyemi_1586/1 -> cfblk60/2
  cfblk185/2(cfblk17) -> cyemi_1586/1
  cyemi_1587/1 -> cfblk61/1
  cfblk27/1 -> cyemi_1587/1
  cfblk38/1 -> cyemi_1588/1, emi_808/1
  cyemi_1590/1 -> cfblk63/1
  cfblk207/1(cfblk2) -> cyemi_1590/1
  cyemi_1592/1 -> cfblk65/1
  cfblk113/1 -> cyemi_1592/1
  cfblk172/3(cfblk11) -> cyemi_1593/1
  cyemi_1594/1 -> cfblk67/1
  cyemi_1595/1 -> cfblk67/2
  cfblk183/2(cfblk12) -> cyemi_1595/1
  cyemi_1597/1 -> cfblk69/1
  cyemi_1598/1 -> cfblk7/1
  cfblk199/2(cfblk11) -> cyemi_1598/1
  cyemi_1599/1 -> cfblk70/1
  cyemi_1600/1 -> cfblk70/2
  cyemi_1601/1 -> cfblk71/1
  cfblk164/3(cfblk14) -> cyemi_1601/1
  cyemi_1602/1 -> cfblk71/2
  cfblk54/1 -> cyemi_1602/1
  cyemi_1603/1 -> cfblk72/1
  cfblk204/2(cfblk12) -> cyemi_1603/1
  cyemi_1604/1 -> cfblk73/1
  cyemi_1605/1 -> cfblk73/2
  cyemi_1606/1 -> cfblk74/1
  cfblk111/1 -> cyemi_1606/1
  cyemi_1607/1 -> cfblk75/1
  cyemi_1608/1 -> cfblk76/1
  cfblk164/4(cfblk15) -> cyemi_1608/1
  cyemi_1610/1 -> cfblk82/1
  cfblk206/1(cfblk2) -> cyemi_1610/1
  cyemi_1611/1 -> cfblk84/1
  cyemi_1614/1 -> cfblk93/1
  cyemi_1575/1 -> cfblk53/1(emi_43)
  cfblk53/1(emi_44) -> cyemi_1613/1, cyemi_27/1
  emi_47/1 -> cfblk53/Action
  emi_47/2 -> emi_45/Action
  emi_48/1 -> emi_47/1
  cyemi_1516/1 -> cfblk256/1(emi_143)
  cfblk256/1(emi_144) -> cyemi_42/1
  emi_147/1 -> cfblk256/Action
  emi_147/2 -> emi_145/Action
  emi_148/1 -> emi_147/1
  cyemi_1612/1 -> cfblk9/1(emi_264)
  cyemi_1613/1 -> cfblk9/2(emi_265)
  cfblk9/1(emi_266) -> emi_708/1, emi_1112/1, cyemi_1526/1
  emi_269/1 -> cfblk9/Action
  emi_269/2 -> emi_267/Action
  emi_270/1 -> emi_269/1
  cyemi_1499/1 -> cfblk240/1(emi_329)
  cfblk240/1(emi_330) -> cyemi_382/1, emi_1448/1
  emi_333/1 -> cfblk240/Action
  emi_333/2 -> emi_331/Action
  emi_334/1 -> emi_333/1
  cyemi_1496/1 -> cfblk239/1(emi_373)
  cfblk239/1(emi_374) -> cyemi_585/1
  emi_377/1 -> cfblk239/Action
  emi_377/2 -> emi_375/Action
  emi_378/1 -> emi_377/1
  cyemi_1506/1 -> cfblk247/1(emi_401)
  cfblk247/1(emi_402) -> cyemi_672/1, emi_744/1, emi_2017/1
  emi_405/1 -> cfblk247/Action
  emi_405/2 -> emi_403/Action
  emi_406/1 -> emi_405/1
  cyemi_1488/1 -> cfblk231/1(emi_436)
  cfblk231/1(emi_437) -> cyemi_671/1
  emi_440/1 -> cfblk231/Action
  emi_440/2 -> emi_438/Action
  emi_441/1 -> emi_440/1
  cyemi_1541/1 -> cfblk29/1(emi_457)
  cyemi_1542/1 -> cfblk29/2(emi_458)
  cfblk29/1(emi_459) -> cyemi_1596/1, cyemi_517/1
  emi_462/1 -> cfblk29/Action
  emi_462/2 -> emi_460/Action
  emi_463/1 -> emi_462/1
  cyemi_1535/1 -> cfblk273/1(emi_465)
  cfblk273/1(emi_466) -> cyemi_11/1, emi_1819/1
  emi_469/1 -> cfblk273/Action
  emi_469/2 -> emi_467/Action
  emi_470/1 -> emi_469/1
  cyemi_1546/1 -> cfblk32/1(emi_480)
  cfblk32/1(emi_481) -> cyemi_1474/1, cfblk100/1
  emi_484/1 -> cfblk32/Action
  emi_484/2 -> emi_482/Action
  emi_485/1 -> emi_484/1
  cyemi_1609/1 -> cfblk8/1(emi_660)
  cfblk8/1(emi_661) -> cyemi_23/1
  emi_664/1 -> cfblk8/Action
  emi_664/2 -> emi_662/Action
  emi_665/1 -> emi_664/1
  cyemi_1474/1 -> cfblk22/1(emi_702)
  cyemi_1475/1 -> cfblk22/2(emi_703)
  cfblk22/1(emi_704) -> cyemi_1524/1, cyemi_1523/1
  emi_707/1 -> cfblk22/Action
  emi_707/2 -> emi_705/Action
  emi_708/1 -> emi_707/1
  cyemi_1588/1 -> cfblk62/1(emi_710)
  cyemi_1589/1 -> cfblk62/2(emi_711)
  cfblk62/1(emi_712) -> cyemi_1591/1, emi_1398/1
  emi_715/1 -> cfblk62/Action
  emi_715/2 -> emi_713/Action
  emi_716/1 -> emi_715/1
  cyemi_1487/1 -> cfblk230/1(emi_739)
  cfblk230/1(emi_740) -> cyemi_406/1
  emi_743/1 -> cfblk230/Action
  emi_743/2 -> emi_741/Action
  emi_744/1 -> emi_743/1
  cyemi_1555/1 -> cfblk39/1(emi_753)
  cfblk39/1(emi_754) -> cyemi_1479/1
  emi_757/1 -> cfblk39/Action
  emi_757/2 -> emi_755/Action
  emi_758/1 -> emi_757/1
  cyemi_7/1 -> cfblk12/1(emi_802)
  cyemi_8/1 -> cfblk12/2(emi_803)
  cfblk12/1(emi_804) -> emi_758/1, cyemi_1263/1, cyemi_1551/1
  emi_807/1 -> cfblk12/Action
  emi_807/2 -> emi_805/Action
  emi_808/1 -> emi_807/1
  cyemi_1547/1 -> cfblk33/1(emi_868)
  cfblk33/1(emi_869) -> cyemi_1311/1
  emi_872/1 -> cfblk33/Action
  emi_872/2 -> emi_870/Action
  emi_873/1 -> emi_872/1
  cyemi_1519/1 -> cfblk259/1(emi_882)
  cfblk259/1(emi_883) -> cyemi_917/1
  emi_886/1 -> cfblk259/Action
  emi_886/2 -> emi_884/Action
  emi_887/1 -> emi_886/1
  cyemi_1564/1 -> cfblk45/1(emi_931)
  cfblk45/1(emi_932) -> emi_873/1, cyemi_770/1
  emi_935/1 -> cfblk45/Action
  emi_935/2 -> emi_933/Action
  emi_936/1 -> emi_935/1
  cyemi_1476/1 -> cfblk220/1(emi_945)
  cfblk220/1(emi_946) -> cyemi_515/1
  emi_949/1 -> cfblk220/Action
  emi_949/2 -> emi_947/Action
  emi_950/1 -> emi_949/1
  cyemi_1593/1 -> cfblk66/1(emi_1008)
  cfblk66/1(emi_1009) -> cyemi_1594/1
  emi_1012/1 -> cfblk66/Action
  emi_1012/2 -> emi_1010/Action
  emi_1013/1 -> emi_1012/1
  cyemi_1558/1 -> cfblk41/1(emi_1036)
  cfblk41/1(emi_1037) -> cyemi_1543/1, cyemi_1489/1
  emi_1040/1 -> cfblk41/Action
  emi_1040/2 -> emi_1038/Action
  emi_1041/1 -> emi_1040/1
  cyemi_1591/1 -> cfblk64/1(emi_1107)
  cfblk64/1(emi_1108) -> cyemi_1507/1
  emi_1111/1 -> cfblk64/Action
  emi_1111/2 -> emi_1109/Action
  emi_1112/1 -> emi_1111/1
  cyemi_1142/1 -> cfblk2/1(emi_1245)
  cfblk2/1(emi_1246) -> cyemi_1600/1, cyemi_1368/1
  emi_1249/1 -> cfblk2/Action
  emi_1249/2 -> emi_1247/Action
  emi_1250/1 -> emi_1249/1
  cyemi_1557/1 -> cfblk40/1(emi_1294)
  cfblk40/1(emi_1295) -> cyemi_1559/1
  emi_1298/1 -> cfblk40/Action
  emi_1298/2 -> emi_1296/Action
  emi_1299/1 -> emi_1298/1
  cyemi_1473/1 -> cfblk219/1(emi_1337)
  cfblk219/1(emi_1338) -> cyemi_36/1
  emi_1341/1 -> cfblk219/Action
  emi_1341/2 -> emi_1339/Action
  emi_1342/1 -> emi_1341/1
  cyemi_1483/1 -> cfblk227/1(emi_1393)
  cfblk227/1(emi_1394) -> cyemi_587/1
  emi_1397/1 -> cfblk227/Action
  emi_1397/2 -> emi_1395/Action
  emi_1398/1 -> emi_1397/1
  cyemi_1468/1 -> cfblk214/1(emi_1443)
  cfblk214/1(emi_1444) -> cyemi_7/1
  emi_1447/1 -> cfblk214/Action
  emi_1447/2 -> emi_1445/Action
  emi_1448/1 -> emi_1447/1
  cyemi_1573/1 -> cfblk52/1(emi_1478)
  cyemi_1574/1 -> cfblk52/2(emi_1479)
  cfblk52/1(emi_1480) -> cyemi_878/1
  emi_1483/1 -> cfblk52/Action
  emi_1483/2 -> emi_1481/Action
  emi_1484/1 -> emi_1483/1
  cyemi_1469/1 -> cfblk215/1(emi_1515)
  cfblk215/1(emi_1516) -> cyemi_1261/1
  emi_1519/1 -> cfblk215/Action
  emi_1519/2 -> emi_1517/Action
  emi_1520/1 -> emi_1519/1
  cyemi_1490/1 -> cfblk233/1(emi_1543)
  cfblk233/1(emi_1544) -> emi_936/1, cyemi_369/1
  emi_1547/1 -> cfblk233/Action
  emi_1547/2 -> emi_1545/Action
  emi_1548/1 -> emi_1547/1
  cyemi_1539/1 -> cfblk277/1(emi_1742)
  cfblk277/1(emi_1743) -> cyemi_1597/1
  emi_1746/1 -> cfblk277/Action
  emi_1746/2 -> emi_1744/Action
  emi_1747/1 -> emi_1746/1
  cyemi_1472/1 -> cfblk218/1(emi_1786)
  cfblk218/1(emi_1787) -> cyemi_329/1
  emi_1790/1 -> cfblk218/Action
  emi_1790/2 -> emi_1788/Action
  emi_1791/1 -> emi_1790/1
  cyemi_1584/1 -> cfblk6/1(emi_1814)
  cfblk6/1(emi_1815) -> cyemi_4/1
  emi_1818/1 -> cfblk6/Action
  emi_1818/2 -> emi_1816/Action
  emi_1819/1 -> emi_1818/1
  cyemi_1529/1 -> cfblk268/1(emi_1878)
  cfblk268/1(emi_1879) -> emi_1041/1, emi_270/1, cyemi_1144/1
  emi_1882/1 -> cfblk268/Action
  emi_1882/2 -> emi_1880/Action
  emi_1883/1 -> emi_1882/1
  cyemi_1515/1 -> cfblk255/1(emi_1913)
  cfblk255/1(emi_1914) -> cyemi_95/1
  emi_1917/1 -> cfblk255/Action
  emi_1917/2 -> emi_1915/Action
  emi_1918/1 -> emi_1917/1
  cyemi_1596/1 -> cfblk68/1(emi_2012)
  cfblk68/1(emi_2013) -> cyemi_1609/1
  emi_2016/1 -> cfblk68/Action
  emi_2016/2 -> emi_2014/Action
  emi_2017/1 -> emi_2016/1

== system sampleModel7293_pp_1_1_mu/cfblk12 ==
  emi_802 : Inport
  emi_803 : Inport  Port=2
  Action Port : ActionPort  ActionType=then
  cfblk12 : Delay  ShowEnablePort=on  SampleTime=1
      settings: InputPortMap=u0,e6
  emi_804 : Outport
  wires:
  emi_802/1 -> cfblk12/1
  emi_803/1 -> cfblk12/2
  cfblk12/1 -> emi_804/1

== system sampleModel7293_pp_1_1_mu/cfblk164 ==
  cfblk1 : Inport
  cfblk10 : Inport  Port=2
  cfblk11 : Inport  Port=3
  cfblk12 : Inport  Port=4
  Action Port : ActionPort  ActionType=then
  cfblk3 : DiscreteIntegrator  SampleTime=-1  OutDataTypeStr=uint16  ICPrevOutput=DiscIntNeverNeededParam  ICPrevScaledInput=DiscIntNeverNeededParam
  cfblk4 : Subsystem  TreatAsAtomicUnit=on
  cfblk5 : simulink/Discrete/Transfer Fcn Real Zero  ZeroZ=0.75  ICPrevInput=0.0  DoSatur=off
      settings: SourceProductName=Simulink  SourceProductBaseCode=SL
  cfblk6 : DiscreteZeroPole  Poles=[0 0.5]  Gain=1  SampleTime=-1
  cfblk7 : Subsystem  TreatAsAtomicUnit=on
  cfblk8 : simulink/Discrete/Transfer Fcn Lead or Lag  PoleZ=0.95  ZeroZ=0.75  ICPrevOutput=0.0  ICPrevInput=0.0  DoSatur=off
      settings: SourceProductName=Simulink  SourceProductBaseCode=SL
  cfblk9 : simulink/Discrete/Transfer Fcn Lead or Lag  PoleZ=0.95  ZeroZ=0.75  ICPrevOutput=0.0  ICPrevInput=0.0  DoSatur=off
      settings: SourceProductName=Simulink  SourceProductBaseCode=SL
  cyemi_43 : DataTypeConversion  OutDataTypeStr=uint16
  cyemi_{44..50} (7 alike) : DataTypeConversion  OutDataTypeStr=double
  emi_1617 : Subsystem  TreatAsAtomicUnit=on
  emi_1619 : If  IfExpression=0 <= u1
  emi_1620 : DataTypeConversion  OutDataTypeStr=uint16
  emi_762 : Subsystem  TreatAsAtomicUnit=on
  emi_764 : If  IfExpression=0 <= u1
  emi_765 : DataTypeConversion  OutDataTypeStr=double
  cfblk2 : Outport
  cfblk13 : Outport  Port=2
  cfblk14 : Outport  Port=3
  cfblk15 : Outport  Port=4
  wires:
  cfblk5/1 -> cfblk13/1
  cfblk1/1 -> cfblk14/1
  cfblk12/1 -> cyemi_48/1, cyemi_49/1
  cfblk3/1 -> cfblk2/1, emi_1620/1
  cyemi_43/1 -> cfblk3/1
  cfblk10/1 -> cyemi_43/1
  cfblk8/1 -> cyemi_44/1
  cyemi_45/1 -> cfblk5/1
  cfblk6/1 -> cyemi_45/1, emi_765/1
  cyemi_46/1 -> cfblk6/1
  cfblk9/1 -> cyemi_46/1
  cfblk11/1 -> cyemi_47/1
  cyemi_49/1 -> cfblk8/1
  cyemi_50/1 -> cfblk9/1
  cyemi_44/1 -> cfblk4/1(emi_760)
  cfblk4/1(emi_761) -> cyemi_50/1
  emi_764/1 -> cfblk4/Action
  emi_764/2 -> emi_762/Action
  emi_765/1 -> emi_764/1
  cyemi_47/1 -> cfblk7/1(emi_1614)
  cyemi_48/1 -> cfblk7/2(emi_1615)
  cfblk7/1(emi_1616) -> cfblk15/1
  emi_1619/1 -> cfblk7/Action
  emi_1619/2 -> emi_1617/Action
  emi_1620/1 -> emi_1619/1

== system sampleModel7293_pp_1_1_mu/cfblk165 ==
  cfblk1 : Inport
  cfblk10 : Inport  Port=2
  cfblk11 : Inport  Port=3
  cfblk12 : Inport  Port=4
  cfblk13 : Inport  Port=5
  Action Port : ActionPort  ActionType=else
  cfblk15 : Subsystem  TreatAsAtomicUnit=on
  cfblk16 : Subsystem  TreatAsAtomicUnit=on
  cfblk17 : Delay
  cfblk3 : simulink/Discrete/Transfer Fcn First Order  PoleZ=0.95  ICPrevOutput=0.0  DoSatur=off
      settings: SourceProductName=Simulink
  cfblk4 : DiscreteZeroPole  Poles=[0 0.5]  Gain=1  SampleTime=-1
  cfblk5 : Subsystem  TreatAsAtomicUnit=on
  cfblk6 : Subsystem  TreatAsAtomicUnit=on
  cfblk7 : DiscreteStateSpace  SampleTime=-1
  cfblk8 : simulink/Continuous/PID Controller  Controller=PID  TimeDomain=Discrete-time  SampleTime=-1  IntegratorMethod=Forward Euler  FilterMethod=Forward Euler  Form=Parallel  UseFilter=on  ControllerParametersSource=internal  P=1  I=1  D=0  N=100  InitialConditionSource=internal  InitialConditionForIntegrator=0  InitialConditionForFilter=0  ExternalReset=none  LimitOutput=off  UpperSaturationLimit=inf  LowerSaturationLimit=-inf  LinearizeAsGain=off  AntiWindupMode=none  Kb=1  TrackingMode=off  Kt=1  PParamMin=[]  PParamMax=[]  IParamMin=[]  IParamMax=[]  DParamMin=[]  DParamMax=[]  NParamMin=[]  NParamMax=[]  KbParamMin=[]  KbParamMax=[]  KtParamMin=[]  KtParamMax=[]  POutMin=[]  POutMax=[]  IOutMin=[]  IOutMax=[]  DOutMin=[]  DOutMax=[]  NOutMin=[]  NOutMax=[]  KbOutMin=[]  KbOutMax=[]  KtOutMin=[]  KtOutMax=[]  IntegratorOutMin=[]  IntegratorOutMax=[]  FilterOutMin=[]  FilterOutMax=[]  SumOutMin=[]  SumOutMax=[]  SumI1OutMin=[]  SumI1OutMax=[]  SumI2OutMin=[]  SumI2OutMax=[]  SumI3OutMin=[]  SumI3OutMax=[]  SumDOutMin=[]  SumDOutMax=[]  SaturationOutMin=[]  SaturationOutMax=[]  IntegratorContinuousStateAttributes=''  IntegratorStateMustResolveToSignalObject=off  IntegratorRTWStateStorageClass=Auto  FilterContinuousStateAttributes=''  FilterStateMustResolveToSignalObject=off  FilterRTWStateStorageClass=Auto  DifferentiatorICPrevScaledInput=0  DifferentiatorOutMin=[]  DifferentiatorOutMax=[]  FilterDiffOutCoefMin=[]  FilterDiffOutCoefMax=[]  SumDenOutMin=[]  SumDenOutMax=[]  SumNumOutMin=[]  SumNumOutMax=[]  ReciprocalOutMin=[]  ReciprocalOutMax=[]  DivideOutMin=[]  DivideOutMax=[]  TunerSelectOption=Transfer Function Based (PID Tuner App)
  cfblk9 : If  SampleTime=1
  cyemi_{56,71,87..94} (10 alike) : DataTypeConversion  OutDataTypeStr=double
  emi_117 : Subsystem  TreatAsAtomicUnit=on
  emi_119 : If  IfExpression=0 <= u1
  emi_120 : DataTypeConversion  OutDataTypeStr=double
  emi_2100 : Subsystem  TreatAsAtomicUnit=on
  emi_2102 : If  IfExpression=0 <= u1
  emi_2103 : DataTypeConversion  OutDataTypeStr=double
  cfblk2 : Outport
  cfblk14 : Outport  Port=2
  wires:
  cfblk3/1 -> cfblk14/1
  cfblk16/1(cfblk2) -> cfblk2/1
  cfblk9/1 -> cfblk15/Action
  cfblk9/2 -> cfblk16/Action
  cyemi_56/1 -> cfblk15/1(cfblk1)
  cfblk13/1 -> cyemi_56/1
  cyemi_71/1 -> cfblk16/1(cfblk1)
  cfblk15/1(cfblk2) -> cyemi_71/1
  cyemi_87/1 -> cfblk17/1
  cfblk16/2(cfblk15) -> cyemi_87/1
  cyemi_88/1 -> cfblk3/1
  cyemi_89/1 -> cfblk4/1
  cfblk11/1 -> cyemi_89/1
  cfblk12/1 -> cyemi_91/1
  cyemi_92/1 -> cfblk7/1
  cfblk17/1 -> cyemi_92/1, emi_2103/1
  cyemi_93/1 -> cfblk8/1
  cfblk10/1 -> cyemi_93/1
  cyemi_94/1 -> cfblk9/1
  cfblk7/1 -> cyemi_94/1
  cyemi_91/1 -> cfblk6/1(emi_115)
  cfblk6/1(emi_116) -> cyemi_90/1
  emi_119/1 -> cfblk6/Action
  emi_119/2 -> emi_117/Action
  emi_120/1 -> emi_119/1
  cyemi_90/1 -> cfblk5/1(emi_2098)
  cfblk5/1(emi_2099) -> emi_120/1, cyemi_88/1
  emi_2102/1 -> cfblk5/Action
  emi_2102/2 -> emi_2100/Action
  emi_2103/1 -> emi_2102/1
